simulink model "JointSpaceControlii"  (Simulink 8.5)
settings: Solver=ode3  StartTime=0.0  StopTime=15  FixedStep=0.05  RelTol=1e-3
values from neighbouring files (symbols this model uses):
  kp = diag([1,1])    [SetupConstants.m]
  kv = diag([2,2])    [SetupConstants.m]
libraries: vrlib x1, simulink x1
settings Model: Creator=Tim Salcudean  LastModifiedBy=tims
settings SolverCC: ZeroCrossControl=DisableAll
settings DataIOCC: ExternalInput=[q0, u]
settings OptimizationCC: InitFltsAndDblsToZero=on
settings DebuggingCC: SaveWithParameterizedLinksMsg=none  SignalResolutionControl=TryResolveAllWithWarning  MaxConsecutiveZCsMsg=warning  MultiTaskDSMMsg=warning  MultiTaskCondExecSysMsg=none  FcnCallInpInsideContextMsg=UseLocalSettings
settings SFSimCC: SimParseCustomCode=off
settings GRTTargetCC: TargetFcnLib=ansi_tfl_tmw.mat

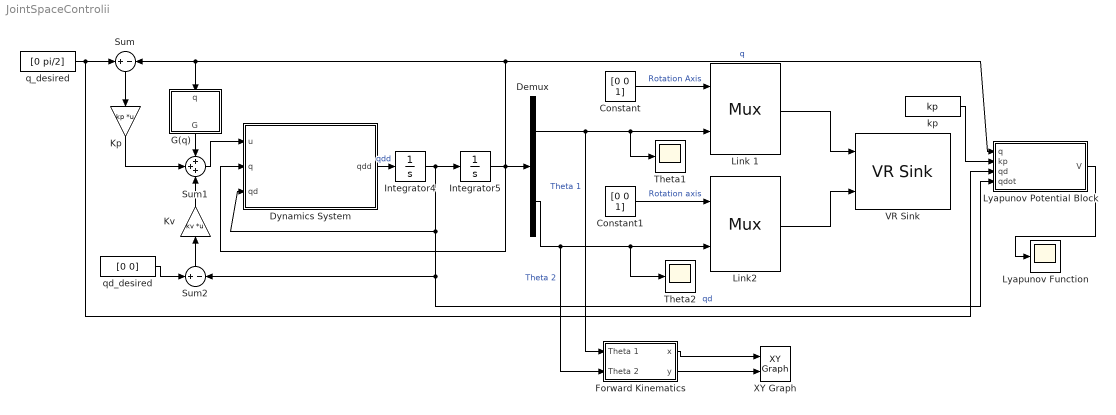
== system JointSpaceControlii ==
  Constant : Constant  Value=[0 0 1]
  Constant1 : Constant  Value=[0 0 1]
  Demux : Demux  Outputs=2
  Dynamics System : MATLAB Function  TreatAsAtomicUnit=on
  Forward Kinematics : Subsystem
  G(q) : MATLAB Function  TreatAsAtomicUnit=on
  Integrator4 : Integrator  InitialCondition=[0;0]
  Integrator5 : Integrator  InitialCondition=[-pi/2 0]
  Kp : Gain  Gain=kp  Multiplication=Matrix(K*u)
  Kv : Gain  Gain=kv  Multiplication=Matrix(K*u)
  Link 1 : Mux  Inputs=2
      settings: DisplayOption=signals
  Link2 : Mux  Inputs=2
      settings: DisplayOption=signals
  Lyapunov Function : Scope
      settings: TickLabels=on  YMin=0  YMax=20  SaveName=ScopeData3
  Lyapunov Potential Block : MATLAB Function  TreatAsAtomicUnit=on
  Sum : Sum  Inputs=+|-
  Sum1 : Sum  Inputs=+++
  Sum2 : Sum  Inputs=+|-
  Theta1 : Scope
  Theta2 : Scope
  VR Sink : vrlib/VR Sink  InstantiateOnLoad=on  SampleTime=-1  ViewEnable=on  RemoteChange=off  RemoteView=off  FieldsWritten=Link1.rotation.4.1.double#Link2.rotation.4.1.double  WorldFileName=HalfScara.WRL  AutoView=off  VideoDimensions=[]  AllowVariableSize=off
  XY Graph : simulink/Sinks/XY Graph  xmin=-2  xmax=2  ymin=-2  ymax=2  st=-1
  kp : Constant  Value=kp
  q_desired : Constant  Value=[0 pi/2]
  qd_desired : Constant  Value=[0 0]
  wires:
  Constant/1 -> Link 1/1  "Rotation Axis"
  Demux/1 -> Link 1/2, Theta1/1, Forward Kinematics/1(Theta 1)  "Theta 1"
  Constant1/1 -> Link2/1  "Rotation axis"
  Demux/2 -> Link2/2, Theta2/1, Forward Kinematics/2(Theta 2)  "Theta 2"
  Link 1/1 -> VR Sink/1
  Link2/1 -> VR Sink/2
  Sum/1 -> Kp/1
  Kv/1 -> Sum1/3
  Sum2/1 -> Kv/1
  q_desired/1 -> Sum/1, Lyapunov Potential Block/3(qd)
  qd_desired/1 -> Sum2/1
  Kp/1 -> Sum1/2
  G(q)/1(G) -> Sum1/1
  Lyapunov Potential Block/1(V) -> Lyapunov Function/1
  kp/1 -> Lyapunov Potential Block/2(kp)
  Forward Kinematics/1(x) -> XY Graph/1
  Forward Kinematics/2(y) -> XY Graph/2
  Dynamics System/1(qdd) -> Integrator4/1  "qdd"
  Integrator5/1 -> Demux/1, Lyapunov Potential Block/1(q), Sum/2, G(q)/1(q), Dynamics System/2(q)  "q"
  Sum1/1 -> Dynamics System/1(u)
  Integrator4/1 -> Dynamics System/3(qd), Sum2/2, Lyapunov Potential Block/4(qdot), Integrator5/1  "qd"

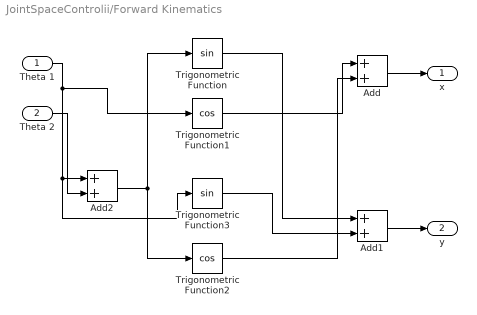
== system JointSpaceControlii/Forward Kinematics ==
  Theta 1 : Inport
  Theta 2 : Inport  Port=2
  Add : Sum
  Add1 : Sum
  Add2 : Sum
  Trigonometric Function : Trigonometry
  Trigonometric Function1 : Trigonometry  Operator=cos
  Trigonometric Function2 : Trigonometry  Operator=cos
  Trigonometric Function3 : Trigonometry
  x : Outport
  y : Outport  Port=2
  wires:
  Add1/1 -> y/1
  Add/1 -> x/1
  Theta 1/1 -> Add2/1, Trigonometric Function3/1, Trigonometric Function1/1
  Theta 2/1 -> Add2/2
  Add2/1 -> Trigonometric Function/1, Trigonometric Function2/1
  Trigonometric Function/1 -> Add1/1
  Trigonometric Function3/1 -> Add1/2
  Trigonometric Function1/1 -> Add/1
  Trigonometric Function2/1 -> Add/2

== matlab function G(q) ==
  data: q input double; G output double
function G = G(q)

g=9.81;
theta1=q(1);
theta2=q(2);
G=[2*g*cos(theta1)+g*cos(theta1+theta2); g*cos(theta1+theta2)];

== matlab function Lyapunov Potential Block ==
  data: q input double; kp input double; V output double; qd input double; qdot input double
function V = Lyapunov(q,kp,qd,qdot)
theta2=q(2);
D=[3+2*cos(theta2) 1+cos(theta2); 1+cos(theta2) 1];
V = (0.5)*(qdot)'*D*(qdot)+0.5*(qd-q)'*kp*(qd-q); %Lyapnov Potential

== matlab function Dynamics System ==
  data: u input double; q input double; qdd output double; qd input double
function qdd  = dynamics(u, q, qd)

g=9.81;
theta1=q(1);
theta2=q(2);
theta1d=qd(1);
theta2d=qd(2);
D=[3+2*cos(theta2) 1+cos(theta2); 1+cos(theta2) 1];
C=[-2*sin(theta2)*theta2d -sin(theta2)*theta2d; sin(theta2)*theta1d 0];
G=[2*g*cos(theta1)+g*cos(theta1+theta2); g*cos(theta1+theta2)];

qdd=inv(D)*(u-G-C*qd);
